simulink model "block_diagram_Shunt"  (R2023b)
settings: Solver=VariableStepAuto  StartTime=0.0  StopTime=10  RelTol=1e-3
values from neighbouring files (symbols this model uses):
  Bm = 0.000001074    (= 1.074e-06)    [setup_params_shunt.m]
  J = 0.21    [setup_params_shunt.m]
  LAA = 0.01    [setup_params_shunt.m]
  LAF = 0.004    [setup_params_shunt.m]
  LFF = 0.167    [setup_params_shunt.m]
  ra = 0.013    [setup_params_shunt.m]
  rf = 1.43    [setup_params_shunt.m]
  Tl = 2.493    [setup_params_shunt.m]
  Va = 24    [setup_params_shunt.m]
settings Model: Creator=Noor  LastModifiedBy=USER
settings SolverCC: AlgebraicLoopSolver=TrustRegion
settings DataIOCC: ReturnWorkspaceOutputs=off
settings DebuggingCC: UnconnectedInputMsg=warning  UnconnectedOutputMsg=warning  UnconnectedLineMsg=warning  ArithmeticOperatorsInVariantConditions=warning
settings ModelReferenceCC: EnableRefExpFcnMdlSchedulingChecks=on
settings SFSimCC: SimUseLocalCustomCode=off  CustomCodeUndefinedFunction=UseInterfaceOnly
settings RTWCC: RTWUseLocalCustomCode=off

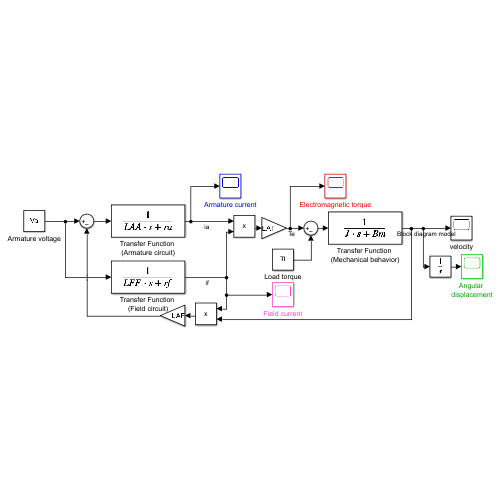
[thumbnail: Simulink's stored preview of the top-level diagram]
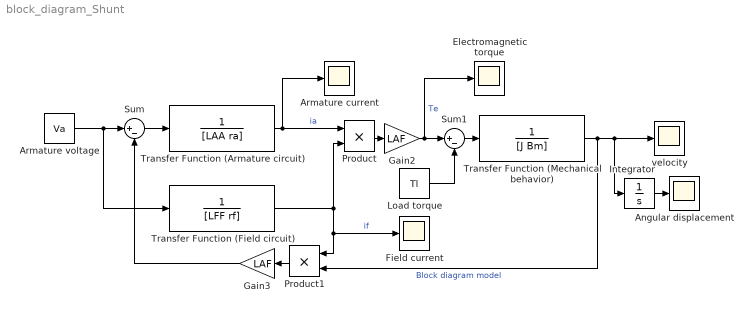
== system block_diagram_Shunt ==
  Angular displacement : Scope
  Armature current : Scope
  Armature voltage : Constant  Value=Va
  Electromagnetic torque : Scope
  Field current : Scope
  Gain2 : Gain  Gain=LAF
  Gain3 : Gain  Gain=LAF
  Integrator : Integrator
  Load torque : Constant  Value=Tl
  Product : Product
  Product1 : Product
  Sum : Sum  Inputs=|+-
  Sum1 : Sum  Inputs=|+-
  Transfer Function (Armature circuit) : TransferFcn  Denominator=[LAA ra]
  Transfer Function (Field circuit) : TransferFcn  Denominator=[LFF rf]
  Transfer Function (Mechanical behavior) : TransferFcn  Denominator=[J Bm]
  velocity : Scope
  wires:
  Transfer Function (Mechanical behavior)/1 -> Product1/2, Integrator/1, velocity/1  "Block diagram model"
  Gain2/1 -> Electromagnetic torque/1, Sum1/1  "Te"
  Gain3/1 -> Sum/2
  Sum/1 -> Transfer Function (Armature circuit)/1
  Armature voltage/1 -> Transfer Function (Field circuit)/1, Sum/1
  Transfer Function (Armature circuit)/1 -> Armature current/1, Product/1  "ia"
  Transfer Function (Field circuit)/1 -> Field current/1, Product1/1, Product/2  "if"
  Product1/1 -> Gain3/1
  Sum1/1 -> Transfer Function (Mechanical behavior)/1
  Product/1 -> Gain2/1
  Integrator/1 -> Angular displacement/1
  Load torque/1 -> Sum1/2
